simulink model "FuelConsDspl_DD"  (R2016b)
settings: configuration reference "CodeGenConfigSet" (kept outside this file)
values from neighbouring files (symbols this model uses):
  FuelConsDspl_bSwtPrs_C = Calibration.Parameter    [init_FuelConsDspl_DD.m]
  FuelConsDspl_O_P_C = Calibration.Parameter    [init_FuelConsDspl_DD.m]
  FuelConsDspl_PwmOut_swtBattCor_C = Calibration.Parameter    [init_FuelConsDspl_DD.m]
  FuelConsDspl_rCnv_CUR = Calibration.Parameter    [init_FuelConsDspl_DD.m]
  FuelConsDspl_rCnv_CURX = Calibration.Parameter    [init_FuelConsDspl_DD.m]
  FuelConsDspl_stEna_C = Calibration.Parameter    [init_FuelConsDspl_DD.m]
  FuelConsDspl_stPsDiaDisbl_C = Calibration.Parameter    [init_FuelConsDspl_DD.m]
  FuelConsDspl_stPsDisbl_C = Calibration.Parameter    [init_FuelConsDspl_DD.m]
  FuelConsDspl_tiPer_C = Calibration.Parameter    [init_FuelConsDspl_DD.m]
undefined symbols (not defined in the file or in its folder): Switch_conv
libraries: simulink x2
settings Model: Creator=liutao  LastModifiedBy=liutao
settings ConfigSetRef: SourceLocation=Base Workspace

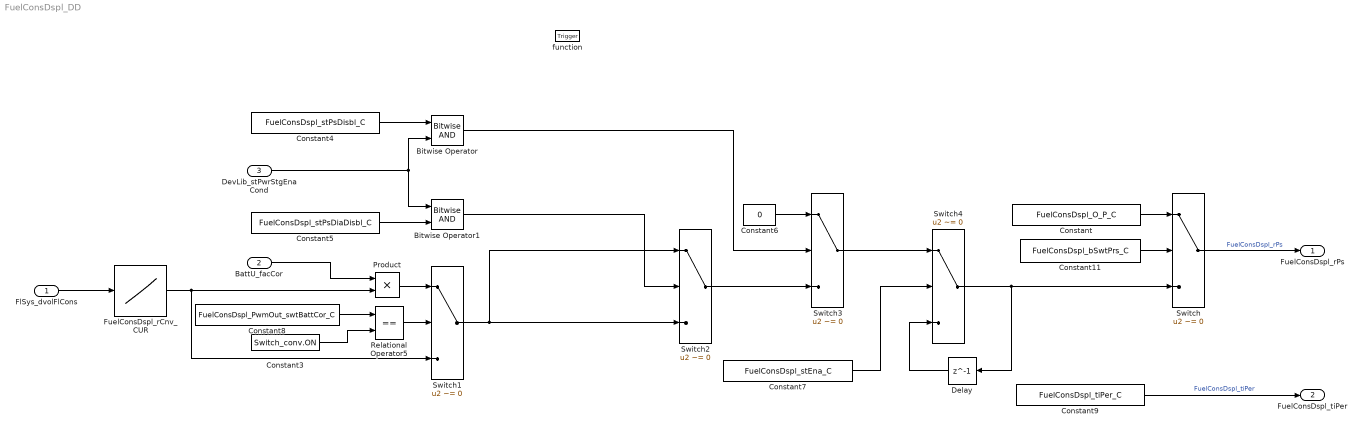
== system FuelConsDspl_DD ==
  FlSys_dvolFlCons : Inport  Tag=L/h  Description=Fuel consumption [l/h]  OutMin=0  OutMax=327  OutDataTypeStr=FlCon_L_h
  BattU_facCor : Inport  Description=Battery correction factor  Port=2  OutMin=-32  OutMax=31.9  OutDataTypeStr=Factor
  DevLib_stPwrStgEnaCond : Inport  Description=Control unit status relevant to power stage deactivation/error diagnosis  Port=3  OutMin=0  OutMax=65535  OutDataTypeStr=State_uint16
  function : TriggerPort  TriggerType=function-call  VariantControl=Variant
  Bitwise Operator : simulink/Logic and Bit Operations/Bitwise Operator  logicop=AND  UseBitMask=off  NumInputPorts=2  BitMask=bin2dec('11011001')  BitMaskRealWorld=Stored Integer
  Bitwise Operator1 : simulink/Logic and Bit Operations/Bitwise Operator  logicop=AND  UseBitMask=off  NumInputPorts=2  BitMask=bin2dec('11011001')  BitMaskRealWorld=Stored Integer
  Constant : Constant  Value=FuelConsDspl_O_P_C
  Constant11 : Constant  Value=FuelConsDspl_bSwtPrs_C  SampleTime=-1
  Constant3 : Constant  Value=Switch_conv.ON  OutDataTypeStr=Inherit: Inherit via back propagation
  Constant4 : Constant  Value=FuelConsDspl_stPsDisbl_C
  Constant5 : Constant  Value=FuelConsDspl_stPsDiaDisbl_C
  Constant6 : Constant  Value=0  OutDataTypeStr=Inherit: Inherit via back propagation
  Constant7 : Constant  Value=FuelConsDspl_stEna_C
  Constant8 : Constant  Value=FuelConsDspl_PwmOut_swtBattCor_C
  Constant9 : Constant  Value=FuelConsDspl_tiPer_C  SampleTime=-1
  Delay : Delay  DelayLength=1  InitialCondition=0
  FuelConsDspl_rCnv_CUR : Lookup_n-D  NumberOfTableDimensions=1  BreakpointsForDimension1=FuelConsDspl_rCnv_CURX  Table=FuelConsDspl_rCnv_CUR  ExtrapMethod=Clip  InternalRulePriority=Speed  RndMeth=Simplest
  Product : Product  OutDataTypeStr=Inherit: Inherit via back propagation  SaturateOnIntegerOverflow=on
  Relational Operator5 : RelationalOperator  Operator===  OutDataTypeStr=boolean  RndMeth=Simplest  InputSameDT=on
  Switch{,2..4} (4 alike) : Switch  Criteria=u2 ~= 0  OutDataTypeStr=Inherit: Inherit via back propagation
  Switch1 : Switch  Criteria=u2 ~= 0
  FuelConsDspl_rPs : Outport  Tag=%  Description=Output to the power stage of fuel consumption PWM output to drive the gauge on the dashboard  OutMin=0  OutMax=100  OutDataTypeStr=DutyCycle_rate
  FuelConsDspl_tiPer : Outport  Tag=us  Description=Class Instance for PWM / Reference value for period duration (small type to limit dynamic range)  Port=2  OutMin=-107374182  OutMax=107374182  OutDataTypeStr=Time_PwmHigh_us
  wires:
  FlSys_dvolFlCons/1 -> FuelConsDspl_rCnv_CUR/1
  FuelConsDspl_rCnv_CUR/1 -> Switch1/3, Product/2
  Constant4/1 -> Bitwise Operator/1
  Product/1 -> Switch1/1
  DevLib_stPwrStgEnaCond/1 -> Bitwise Operator1/1, Bitwise Operator/2
  Constant5/1 -> Bitwise Operator1/2
  Switch1/1 -> Switch2/3, Switch2/1
  Switch2/1 -> Switch3/3
  Constant6/1 -> Switch3/1
  Switch4/1 -> Delay/1, Switch/3
  BattU_facCor/1 -> Product/1
  Bitwise Operator1/1 -> Switch2/2
  Bitwise Operator/1 -> Switch3/2
  Switch3/1 -> Switch4/1
  Constant7/1 -> Switch4/2
  Constant11/1 -> Switch/2
  Switch/1 -> FuelConsDspl_rPs/1  "FuelConsDspl_rPs"
  Constant/1 -> Switch/1
  Delay/1 -> Switch4/3
  Constant3/1 -> Relational Operator5/2
  Relational Operator5/1 -> Switch1/2
  Constant8/1 -> Relational Operator5/1
  Constant9/1 -> FuelConsDspl_tiPer/1  "FuelConsDspl_tiPer"
